simulink model "single_phase_fw"  (Simulink 6.1)
settings: Solver=ode23tb  StartTime=0.0  StopTime=0.1  MaxStep=1e-4  RelTol=1e-3  AbsTol=.01
libraries: powerlib x9
settings Model: LastModifiedBy=ThinkPad
settings DebuggingCC: SolverPrmCheckMsg=warning

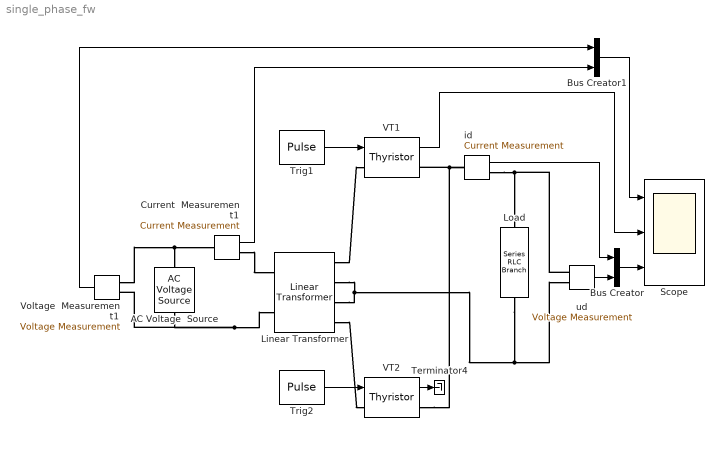
== system single_phase_fw ==
  AC Voltage  Source : powerlib/Electrical Sources/AC Voltage Source  Orientation=up  Amplitude=100  Phase=0  Frequency=50  SampleTime=0  Measurements=None
  Bus Creator : BusCreator  DialogController=Simulink.DDGSource_Bus  Inputs=2
  Bus Creator1 : BusCreator  DialogController=Simulink.DDGSource_Bus  Inputs=2
  Current  Measurement1 : powerlib/Measurements/Current Measurement  PhasorSimulation=off  OutputType=Complex  PSBequivalent=0
  Linear Transformer : powerlib/Elements/Linear Transformer  PhysicalDomain=powersysdomain  SubClassName=unknown  LeftPortType=p1  RightPortType=p1  LConnTagsString=a|b  RConnTagsString=A|B|C|D  NominalPower=[ 10000 50 ]  winding1="[ 100  0.001  0.01 ]"  winding2="[ 100  0.001  0.01 ]"  ThreeWindings=on  winding3="[ 100  0.001  0.01 ]"  RmLm=[ 500 500 ]  Measurements=None
  Load : powerlib/Elements/Series RLC Branch  Orientation=down  PhysicalDomain=powersysdomain  SubClassName=unknown  LeftPortType=p1  RightPortType=p1  LConnTagsString=__new0  RConnTagsString=__new0  Resistance=2  Inductance=0  Capacitance=inf  Measurements=None
  Scope : Scope  NumInputPorts=3
      settings: TimeRange=0.1  YMin=-100~-200~0  YMax=100~200~100  Decimation=5  SampleInput=on  SampleTime=1e-4
  Terminator4 : Terminator
  Trig1 : DiscretePulseGenerator  PulseType=Time based  Amplitude=10  Period=0.02  PulseWidth=5  PhaseDelay=0.0025
  Trig2 : DiscretePulseGenerator  PulseType=Time based  Amplitude=10  Period=0.02  PulseWidth=5  PhaseDelay=0.0125
  VT1 : powerlib/Power Electronics/Thyristor  Ron=0.01  Lon=0  Vf=0.8  IC=0  Rs=1000  Cs=100e-9  Measurements=on
  VT2 : powerlib/Power Electronics/Thyristor  Ron=0.01  Lon=0  Vf=0.8  IC=0  Rs=1000  Cs=100e-9  Measurements=on
  Voltage  Measurement1 : powerlib/Measurements/Voltage Measurement  Orientation=left  PhasorSimulation=off  OutputType=Complex  PSBequivalent=0
  id : powerlib/Measurements/Current Measurement  PhasorSimulation=off  OutputType=Complex  PSBequivalent=0
  ud : powerlib/Measurements/Voltage Measurement  PhasorSimulation=off  OutputType=Complex  PSBequivalent=0
  wires:
  Trig1/1 -> VT1/1
  VT1/1 -> Scope/2
  ud/1 -> Bus Creator/2
  Bus Creator/1 -> Scope/3
  id/1 -> Bus Creator/1
  Trig2/1 -> VT2/1
  Bus Creator1/1 -> Scope/1
  Voltage  Measurement1/1 -> Bus Creator1/1
  Current  Measurement1/1 -> Bus Creator1/2
  VT2/1 -> Terminator4/1
  connections:
  ud/LConn1 -- Load/LConn1 -- id/RConn1
  id/LConn1 -- VT1/RConn1 -- VT2/RConn1
  Linear Transformer/RConn2 -- Load/RConn1 -- ud/LConn2 -- Linear Transformer/RConn3
  Voltage  Measurement1/LConn1 -- AC Voltage  Source/RConn1 -- Current  Measurement1/LConn1
  AC Voltage  Source/LConn1 -- Voltage  Measurement1/LConn2 -- Linear Transformer/LConn2
  Linear Transformer/RConn1 -- VT1/LConn1
  Linear Transformer/RConn4 -- VT2/LConn1
  Current  Measurement1/RConn1 -- Linear Transformer/LConn1
